simulink model "questao7"  (R2023a)
settings: Solver=VariableStepAuto  StartTime=0.0  StopTime=160  FixedStep=1  MaxStep=0.1  RelTol=1e-3
values from neighbouring files (symbols this model uses):
  B = 0.1    [trab_controle.m]
  J = 1    [trab_controle.m]
  Km = 1/3    (= 0.333333333333)    [trab_controle.m]
  L = 0.5    [trab_controle.m]
  R = 10    [trab_controle.m]
settings Model: Creator=franz  LastModifiedBy=franz

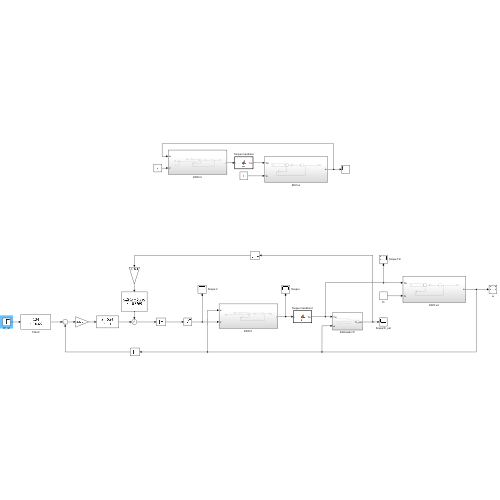
[thumbnail: Simulink's stored preview of the top-level diagram]
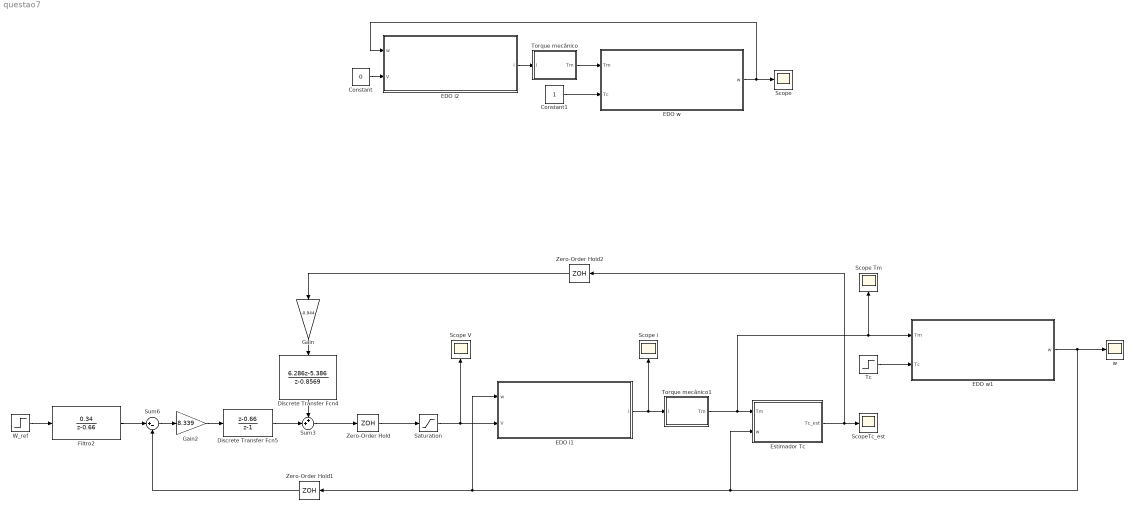
== system questao7 ==
  Constant : Constant  Value=0
  Constant1 : Constant
  Discrete Transfer Fcn4 : DiscreteTransferFcn  Numerator=[6.286 -5.386]  Denominator=[1 -0.8569]
  Discrete Transfer Fcn5 : DiscreteTransferFcn  Numerator=[1 -0.66]  Denominator=[1 -1]
  EDO i1 : Subsystem
  EDO i2 : Subsystem
  EDO w : Subsystem
  EDO w1 : Subsystem
  Estimador Tc : Subsystem
  Filtro2 : DiscreteTransferFcn  Numerator=[0 0.34]  Denominator=[1 -0.66]
  Gain : Gain  Gain=-0.944
  Gain2 : Gain  Gain=8.339
  Saturation : Saturate  UpperLimit=40  LowerLimit=-40
  Scope : Scope
  Scope Tm : Scope
  Scope V : Scope
  Scope i : Scope
  ScopeTc_est : Scope
  Sum3 : Sum  Inputs=++|
  Sum6 : Sum  Inputs=|+-
  Tc : Step  Time=100  Before=0.5  After=1.5  SampleTime=0
  Torque mecânico : MATLAB Function  TreatAsAtomicUnit=on
  Torque mecânico1 : MATLAB Function  TreatAsAtomicUnit=on
  W_ref : Step  Time=80  Before=25  After=27  SampleTime=0
  Zero-Order Hold : ZeroOrderHold  SampleTime=-1
  Zero-Order Hold1 : ZeroOrderHold  SampleTime=-1
  Zero-Order Hold2 : ZeroOrderHold  SampleTime=-1
  w : Scope
  wires:
  Discrete Transfer Fcn5/1 -> Sum3/2
  Filtro2/1 -> Sum6/1
  Discrete Transfer Fcn4/1 -> Sum3/1
  Sum6/1 -> Gain2/1
  Gain2/1 -> Discrete Transfer Fcn5/1
  W_ref/1 -> Filtro2/1
  Estimador Tc/1(Tc_est) -> ScopeTc_est/1, Zero-Order Hold2/1
  Constant/1 -> EDO i2/2(V)
  EDO i2/1(i) -> Torque mecânico/1(i)
  Torque mecânico/1(Tm) -> EDO w/1(Tm)
  Constant1/1 -> EDO w/2(Tc)
  EDO w/1(w) -> Scope/1, EDO i2/1(w)
  EDO i1/1(i) -> Torque mecânico1/1(i), Scope i/1
  Torque mecânico1/1(Tm) -> Estimador Tc/1(Tm), EDO w1/1(Tm), Scope Tm/1
  Tc/1 -> EDO w1/2(Tc)
  EDO w1/1(w) -> Estimador Tc/2(w), Zero-Order Hold1/1, EDO i1/1(w), w/1
  Sum3/1 -> Zero-Order Hold/1
  Gain/1 -> Discrete Transfer Fcn4/1
  Zero-Order Hold/1 -> Saturation/1
  Zero-Order Hold1/1 -> Sum6/2
  Zero-Order Hold2/1 -> Gain/1
  Saturation/1 -> EDO i1/2(V), Scope V/1

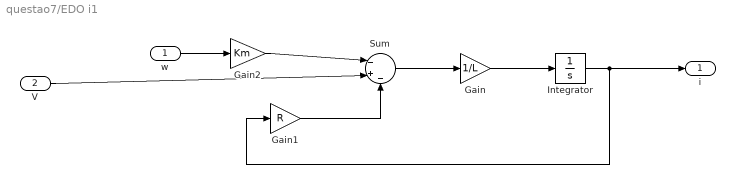
== system questao7/EDO i1 ==
  w : Inport
  V : Inport  Port=2
  Gain : Gain  Gain=1/L
  Gain1 : Gain  Gain=R
  Gain2 : Gain  Gain=Km
  Integrator : Integrator
  Sum : Sum  Inputs=|-+-
  i : Outport
  wires:
  Gain1/1 -> Sum/3
  Integrator/1 -> i/1, Gain1/1
  Gain/1 -> Integrator/1
  Sum/1 -> Gain/1
  w/1 -> Gain2/1
  Gain2/1 -> Sum/1
  V/1 -> Sum/2

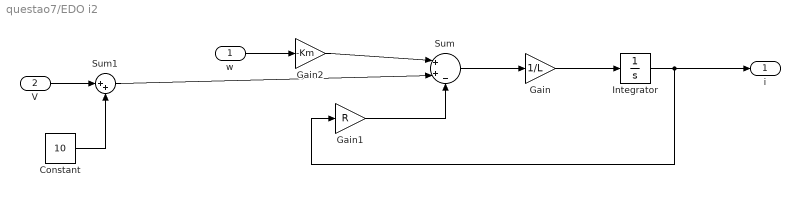
== system questao7/EDO i2 ==
  w : Inport
  V : Inport  Port=2
  Constant : Constant  Value=10
  Gain : Gain  Gain=1/L
  Gain1 : Gain  Gain=R
  Gain2 : Gain  Gain=-Km
  Integrator : Integrator  InitialCondition=0.5708
  Sum : Sum  Inputs=|++-
  Sum1 : Sum  Inputs=|++
  i : Outport
  wires:
  Constant/1 -> Sum1/2
  Sum1/1 -> Sum/2
  V/1 -> Sum1/1
  Gain2/1 -> Sum/1
  w/1 -> Gain2/1
  Sum/1 -> Gain/1
  Gain/1 -> Integrator/1
  Integrator/1 -> Gain1/1, i/1
  Gain1/1 -> Sum/3

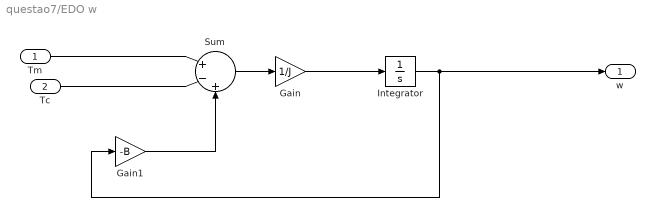
== system questao7/EDO w ==
  Tm : Inport
  Tc : Inport  Port=2
  Gain : Gain  Gain=1/J
  Gain1 : Gain  Gain=-B
  Integrator : Integrator  InitialCondition=12.8766
  Sum : Sum  Inputs=|+-+
  w : Outport
  wires:
  Integrator/1 -> w/1, Gain1/1
  Gain1/1 -> Sum/3
  Gain/1 -> Integrator/1
  Tc/1 -> Sum/2
  Sum/1 -> Gain/1
  Tm/1 -> Sum/1

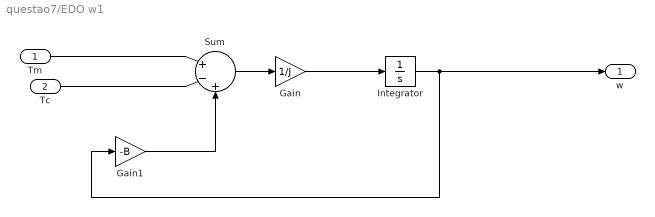
== system questao7/EDO w1 ==
  Tm : Inport
  Tc : Inport  Port=2
  Gain : Gain  Gain=1/J
  Gain1 : Gain  Gain=-B
  Integrator : Integrator
  Sum : Sum  Inputs=|+-+
  w : Outport
  wires:
  Tm/1 -> Sum/1
  Sum/1 -> Gain/1
  Tc/1 -> Sum/2
  Gain/1 -> Integrator/1
  Gain1/1 -> Sum/3
  Integrator/1 -> Gain1/1, w/1

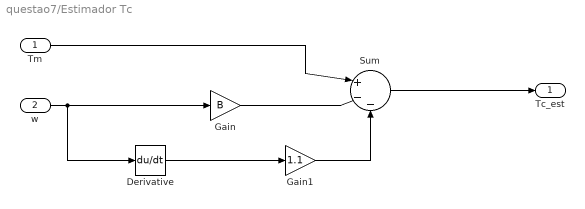
== system questao7/Estimador Tc ==
  Tm : Inport
  w : Inport  Port=2
  Derivative : Derivative
  Gain : Gain  Gain=B
  Gain1 : Gain  Gain=1.1
  Sum : Sum  Inputs=|+--
  Tc_est : Outport
  wires:
  w/1 -> Derivative/1, Gain/1
  Gain/1 -> Sum/2
  Tm/1 -> Sum/1
  Derivative/1 -> Gain1/1
  Gain1/1 -> Sum/3
  Sum/1 -> Tc_est/1

== matlab function questao7/Torque mecânico1 ==
  data: i input; Tm output
function Tm = fcn(i)

if i >= 0
    torque_m = 5.26*(1 - exp(-i));
else
    torque_m = -5.26*(1 - exp(i));
end
Tm = torque_m;

== matlab function questao7/Torque mecânico ==
  data: i input; Tm output
function Tm = fcn(i)

if i >= 0
    torque_m = 5.26*(1 - exp(-i));
else
    torque_m = -5.26*(1 - exp(i));
end


Tm = torque_m;
